simulink model "DT_UDE"  (R2020a)
settings: Solver=FixedStepAuto  StartTime=0.0  StopTime=tstop  FixedStep=tstep  RelTol=1e-3
values from neighbouring files (symbols this model uses):
  eic = xic - xmic    [data.m]
  K = dlqr(F_n, G_n, Q, R)    [data.m]
  udic = (-tstep/T)*pinv(G_n)*eic    [data.m]
  xic = [-2; 1]    [data.m]
  xmic = [-3; -2]    [data.m]
settings Model: Creator=Ram Padmanabhan  LastModifiedBy=Ram Padmanabhan
settings DataIOCC: SaveOutput=off  SignalLogging=off  DSMLogging=off  SaveTime=off  ReturnWorkspaceOutputs=off

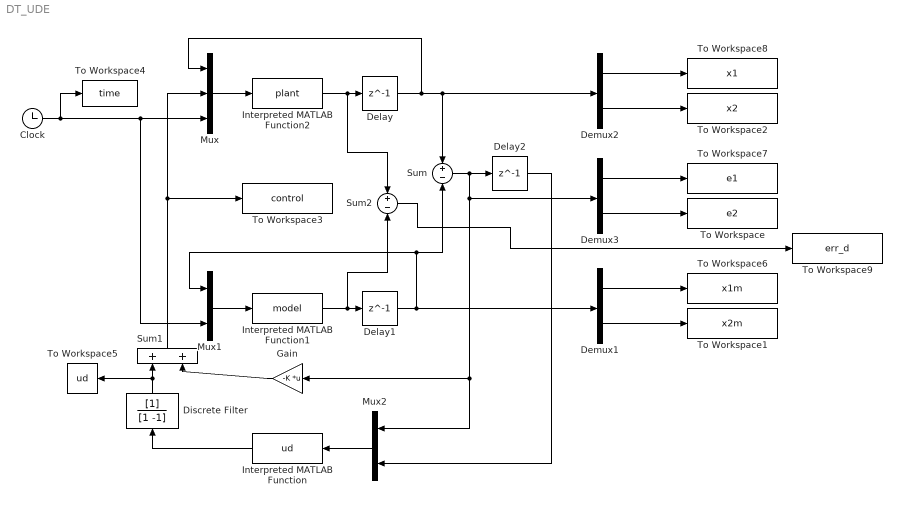
== system DT_UDE ==
  Clock : Clock
  Delay : Delay  DelayLength=1  InitialCondition=xic
  Delay1 : Delay  DelayLength=1  InitialCondition=xmic
  Delay2 : Delay  DelayLength=1  InitialCondition=eic
  Demux1 : Demux  Outputs=2
  Demux2 : Demux  Outputs=2
  Demux3 : Demux  Outputs=2
  Discrete Filter : DiscreteFilter  Denominator=[1 -1]  InitialStates=udic
  Gain : Gain  Gain=-K  Multiplication=Matrix(K*u)
  Interpreted MATLAB Function : MATLABFcn  MATLABFcn=ud  OutputDimensions=1
  Interpreted MATLAB Function1 : MATLABFcn  MATLABFcn=model  OutputDimensions=2
  Interpreted MATLAB Function2 : MATLABFcn  MATLABFcn=plant  OutputDimensions=2
  Mux : Mux  Inputs=3
  Mux1 : Mux  Inputs=2
  Mux2 : Mux  Inputs=2
  Sum : Sum  Inputs=+-
  Sum1 : Sum
  Sum2 : Sum  Inputs=+-
  To Workspace : ToWorkspace  VariableName=e2  SampleTime=-1
  To Workspace1 : ToWorkspace  VariableName=x2m  SampleTime=-1
  To Workspace2 : ToWorkspace  VariableName=x2  SampleTime=-1
  To Workspace3 : ToWorkspace  VariableName=control  SampleTime=-1
  To Workspace4 : ToWorkspace  VariableName=time  SampleTime=-1
  To Workspace5 : ToWorkspace  VariableName=ud  SampleTime=-1
  To Workspace6 : ToWorkspace  VariableName=x1m  SampleTime=-1
  To Workspace7 : ToWorkspace  VariableName=e1  SampleTime=-1
  To Workspace8 : ToWorkspace  VariableName=x1  SampleTime=-1
  To Workspace9 : ToWorkspace  VariableName=err_d  SampleTime=-1
  wires:
  Interpreted MATLAB Function2/1 -> Sum2/1, Delay/1
  Interpreted MATLAB Function1/1 -> Sum2/2, Delay1/1
  Mux/1 -> Interpreted MATLAB Function2/1
  Delay/1 -> Sum/1, Demux2/1, Mux/1
  Clock/1 -> Mux/3, Mux1/2, To Workspace4/1
  Mux1/1 -> Interpreted MATLAB Function1/1
  Delay1/1 -> Sum/2, Mux1/1, Demux1/1
  Sum/1 -> Delay2/1, Gain/1, Mux2/1, Demux3/1
  Mux2/1 -> Interpreted MATLAB Function/1
  Delay2/1 -> Mux2/2
  Interpreted MATLAB Function/1 -> Discrete Filter/1
  Sum1/1 -> Mux/2, To Workspace3/1
  Demux2/1 -> To Workspace8/1
  Demux2/2 -> To Workspace2/1
  Demux3/1 -> To Workspace7/1
  Demux3/2 -> To Workspace/1
  Demux1/1 -> To Workspace6/1
  Demux1/2 -> To Workspace1/1
  Gain/1 -> Sum1/2
  Discrete Filter/1 -> To Workspace5/1, Sum1/1
  Sum2/1 -> To Workspace9/1
